simulink model "Ventilator_Controller"  (R2019b)
settings: Solver=ode23tb  StartTime=0  StopTime=1000  FixedStep=0.001  MaxStep=time_step_new  RelTol=0.01  EnableMultiTasking=on
values from neighbouring files (symbols this model uses):
  A = 20.9    [Gas_Exchange_IC.m]    (also in getPneumonia.m = (LF1-LF2)/(1-exp(Rresolve*(t2(end)-t2(1)))))
  a1 = 0.3836    [Dissociation_Spencer_IC.m]    (also in Gas_Exchange_IC.m; Respiratory_IC.m)
  a2 = 1.819    [Dissociation_Spencer_IC.m]    (also in Gas_Exchange_IC.m; Respiratory_IC.m)
  alpha1 = 0.02598    [Dissociation_Spencer_IC.m]    (also in Gas_Exchange_IC.m; Respiratory_IC.m)
  alpha2 = 0.05591    [Dissociation_Spencer_IC.m]    (also in Gas_Exchange_IC.m; Respiratory_IC.m)
  B = 92.8    [Gas_Exchange_IC.m]    (also in getPneumonia.m = LungFunction(end)-A)
  beta1 = 0.012275    [Dissociation_Spencer_IC.m]    (also in Gas_Exchange_IC.m; Respiratory_IC.m)
  beta2 = 0.03255    [Dissociation_Spencer_IC.m]    (also in Gas_Exchange_IC.m; Respiratory_IC.m)
  C = 10570    [Gas_Exchange_IC.m]
  C1 = 9    [Dissociation_Spencer_IC.m]    (also in Gas_Exchange_IC.m; Respiratory_IC.m)
  C2 = 87.00    (= 87)    [Dissociation_Spencer_IC.m]    (also in Gas_Exchange_IC.m; Respiratory_IC.m)
  Circadian_Period = 24    [Respiratory_IC.m]    (also in State_UA_Khoo_IC.m)
  CvCO2IC = 0.5116    [Body_Khoo_IC.m]    (also in Gas_Exchange_IC.m; Respiratory_IC.m = 0.5247)
  CvO2IC = 0.1672    [Body_Khoo_IC.m]    (also in Gas_Exchange_IC.m; Respiratory_IC.m = 0.1639)
  D = -5.251    [Gas_Exchange_IC.m]
  Dead1CO2IC = 0.1020    (= 0.102)    [Dead_Space_Khoo_IC.m]    (also in Gas_Exchange_IC.m; Respiratory_IC.m = 39.5616)
  Dead1O2IC = 149.8824    [Dead_Space_Khoo_IC.m]    (also in Gas_Exchange_IC.m; Respiratory_IC.m = 104.3637)
  Dead2CO2IC = 0.5274    [Dead_Space_Khoo_IC.m]    (also in Gas_Exchange_IC.m; Respiratory_IC.m = 39.6736)
  Dead2O2IC = 149.3923    [Dead_Space_Khoo_IC.m]    (also in Gas_Exchange_IC.m; Respiratory_IC.m = 104.2258)
  Dead3CO2IC = 2.2996    [Dead_Space_Khoo_IC.m]    (also in Gas_Exchange_IC.m; Respiratory_IC.m = 39.8127)
  Dead3O2IC = 147.3503    [Dead_Space_Khoo_IC.m]    (also in Gas_Exchange_IC.m; Respiratory_IC.m = 104.0505)
  Dead4CO2IC = 8.2293    [Dead_Space_Khoo_IC.m]    (also in Gas_Exchange_IC.m; Respiratory_IC.m = 40.0061)
  Dead4O2IC = 140.5179    [Dead_Space_Khoo_IC.m]    (also in Gas_Exchange_IC.m; Respiratory_IC.m = 103.8005)
  Dead5CO2IC = 22.0757    [Dead_Space_Khoo_IC.m]    (also in Gas_Exchange_IC.m; Respiratory_IC.m = 40.3359)
  Dead5O2IC = 124.5641    [Dead_Space_Khoo_IC.m]    (also in Gas_Exchange_IC.m; Respiratory_IC.m = 103.3579)
  DtotalIC = 0.3    [NeuroMuscular_IC.m]    (also in Respiratory_IC.m = 0.32)
  E_CW = 5    [Pleural_Schuessler_IC.m]    (also in Pmus_Flow_Younes_IC.m; Resp_Mech_IC.m; Respiratory_IC.m)
  E_L = 5    [Pleural_Schuessler_IC.m]    (also in Pmus_Flow_Younes_IC.m; Resp_Mech_IC.m; Respiratory_IC.m)
  fc = 0.4/60    (= 0.00666666666667)    [Respiratory_IC.m]    (also in State_UA_Khoo_IC.m)
  fcs_max = 47.78    [Cardiovascular_IC.m]    (also in Reflex_Ursino_IC.m)
  fcs_min = 2.52    [Cardiovascular_IC.m]    (also in Reflex_Ursino_IC.m)
  fcs_zero = 25    [Respiratory_IC.m]
  FlowIC = 0    [Pmus_Flow_Younes_IC.m]    (also in Resp_Mech_IC.m; Respiratory_IC.m)
  fp_inf = 6.3    [Respiratory_IC.m]
  fp_zero = 3.2    [Respiratory_IC.m]
  fs_inf = 2.10    (= 2.1)    [Respiratory_IC.m]
  fs_zero = 16.11    [Respiratory_IC.m]
  ftbs_min = 0.1    [Cardiovascular_IC.m]    (also in SA_Node_Ursino_IC.m)
  gc = 0.008/60    (= 0.000133333333333)    [Respiratory_IC.m]    (also in State_UA_Khoo_IC.m)
  h = 0.0183    [Brain_Khoo_IC.m]    (also in Gas_Exchange_IC.m; Respiratory_IC.m)
  HP_basal = 0.58    [Cardiovascular_IC.m]    (also in SA_Node_Ursino_IC.m)
  Ic = 45    [Gas_Exchange_IC.m]    (also in Respiratory_IC.m; Vent_Drive_Khoo_IC.m)
  IpCO2 = 38    [Gas_Exchange_IC.m]    (also in Respiratory_IC.m; Vent_Drive_Khoo_IC.m)
  IpO2 = 102.4    [Gas_Exchange_IC.m]    (also in Respiratory_IC.m; Vent_Drive_Khoo_IC.m)
  K1 = 13    [Dissociation_Spencer_IC.m]    (also in Gas_Exchange_IC.m; Respiratory_IC.m)
  K2 = 194.4    [Dissociation_Spencer_IC.m]    (also in Gas_Exchange_IC.m; Respiratory_IC.m)
  k_cs = 11.758    [Cardiovascular_IC.m]    (also in Reflex_Ursino_IC.m)
  k_p = 7.06    [Respiratory_IC.m]
  k_s = 0.07    [Respiratory_IC.m]
  lambda = 863    [Gas_Exchange_IC.m]    (also in Lungs_Khoo_IC.m; Respiratory_IC.m)
  Mech_Vent_pressure = 17    [Mech_vent_test.m]
  MRbCO2 = 0.0517    [Brain_Khoo_IC.m]    (also in Gas_Exchange_IC.m; Respiratory_IC.m)
  MRCO2 = 0.0033    [Body_Khoo_IC.m]    (also in Gas_Exchange_IC.m; Respiratory_IC.m)
  MRO2 = 0.0038    [Body_Khoo_IC.m]    (also in Gas_Exchange_IC.m; Respiratory_IC.m)
  NM_block_gain = 1    [Mech_vent_test.m]
  PACO2_delayIC = 39.6041    [Cardio_Mix_Lange_IC.m]    (also in Gas_Exchange_IC.m; Respiratory_IC.m = 40.4448)
  PaCO2firstIC = 0.2150    (= 0.215)    [Cardio_Mix_Lange_IC.m]    (also in Gas_Exchange_IC.m; Respiratory_IC.m = -0.2465)
  PACO2IC = 37.1484    [Gas_Exchange_IC.m]    (also in Lungs_Khoo_IC.m; Respiratory_IC.m = 40.9432)
  PaCO2secondIC = 38.4577    [Cardio_Mix_Lange_IC.m]    (also in Gas_Exchange_IC.m; Respiratory_IC.m = 40.3928)
  PAO2_delayIC = 103.8436    [Cardio_Mix_Lange_IC.m]    (also in Gas_Exchange_IC.m; Respiratory_IC.m = 103.1223)
  PaO2firstIC = -0.2838    [Cardio_Mix_Lange_IC.m]    (also in Gas_Exchange_IC.m; Respiratory_IC.m = 0.3557)
  PAO2IC = 107.1983    [Gas_Exchange_IC.m]    (also in Lungs_Khoo_IC.m; Respiratory_IC.m = 102.5153)
  PaO2secondIC = 105.4828    [Cardio_Mix_Lange_IC.m]    (also in Gas_Exchange_IC.m; Respiratory_IC.m = 103.1435)
  PbCO2IC = 48.2858    [Brain_Khoo_IC.m]    (also in Gas_Exchange_IC.m; Respiratory_IC.m = 48.5383)
  PICO2 = 0    [Dead_Space_Khoo_IC.m]    (also in Gas_Exchange_IC.m; Respiratory_IC.m)
  PICO2_change = 0    [Respiratory_IC.m]
  PIO2 = 150    [Dead_Space_Khoo_IC.m]    (also in Gas_Exchange_IC.m; Respiratory_IC.m)
  PIO2_change = -90    [Mech_vent_test.m]    (also in Respiratory_IC.m = 0)
  Pn = 90    [Cardiovascular_IC.m]    (also in Reflex_Ursino_IC.m)
  Pt_frcIC1 = 0    [Pmus_Flow_Younes_IC.m]    (also in Resp_Mech_IC.m; Respiratory_IC.m)
  Pt_frcIC2 = 0    [Pmus_Flow_Younes_IC.m]    (also in Resp_Mech_IC.m; Respiratory_IC.m)
  QdBo = 0.8333    [Brain_Khoo_IC.m]    (also in Gas_Exchange_IC.m; Respiratory_IC.m)
  R_AW = 1.27    [Pleural_Schuessler_IC.m]    (also in Pmus_Flow_Younes_IC.m; Resp_Mech_IC.m; Respiratory_IC.m)
  R_CW = 1.03    [Pleural_Schuessler_IC.m]    (also in Pmus_Flow_Younes_IC.m; Resp_Mech_IC.m; Respiratory_IC.m)
  R_L = 1.69    [Pleural_Schuessler_IC.m]    (also in Pmus_Flow_Younes_IC.m; Resp_Mech_IC.m; Respiratory_IC.m)
  RC = 0.06    [Pleural_Schuessler_IC.m]    (also in Pmus_Flow_Younes_IC.m; Resp_Mech_IC.m; Respiratory_IC.m)
  rc = 0.2/60    (= 0.00333333333333)    [Respiratory_IC.m]    (also in State_UA_Khoo_IC.m)
  SbCO2 = 0.3600    (= 0.36)    [Brain_Khoo_IC.m]    (also in Gas_Exchange_IC.m; Respiratory_IC.m)
  SCO2 = 0.0043    [Brain_Khoo_IC.m]    (also in Gas_Exchange_IC.m; Respiratory_IC.m)
  SWAo = 0.007    [Respiratory_IC.m]    (also in State_UA_Khoo_IC.m)
  T1 = 1    [Cardio_Mix_Lange_IC.m]    (also in Gas_Exchange_IC.m; Respiratory_IC.m)
  T2 = 2    [Cardio_Mix_Lange_IC.m]    (also in Gas_Exchange_IC.m; Respiratory_IC.m)
  t_CO2_duration = 0    [Respiratory_IC.m]
  t_CO2_start = 0    [Respiratory_IC.m]
  t_end_new = 4*24*60*60    (= 345600)    [Mech_vent_test.m]
  t_end_UA = 0    [Respiratory_IC.m]    (also in State_UA_Khoo_IC.m)
  t_Mech_Vent_duration = 0    [Mech_vent_test.m]
  t_Mech_Vent_start = 0    [Mech_vent_test.m]
  t_Mueller_duration = 0    [NeuroMuscular_IC.m]
  t_Mueller_insp = 0    [NeuroMuscular_IC.m]
  t_Mueller_start = 0    [NeuroMuscular_IC.m]
  t_NM_block_duration = 0    [Mech_vent_test.m]
  t_NM_block_start = 0    [Mech_vent_test.m]
  t_O2_duration = 0    [Mech_vent_test.m]    (also in Respiratory_IC.m)
  t_O2_start = 0    [Mech_vent_test.m]    (also in Respiratory_IC.m)
  t_start_new = 0    [Mech_vent_test.m]
  t_start_UA = 0    [Respiratory_IC.m]    (also in State_UA_Khoo_IC.m)
  t_valsalva_duration = 0    [NeuroMuscular_IC.m]
  t_valsalva_insp = 0    [NeuroMuscular_IC.m]
  t_valsalva_start = 0    [NeuroMuscular_IC.m]
  time_step = time_step    [acquire_data.m]    (also in acquire_data_save.m)
  VC = 5    [Pmus_Flow_Younes_IC.m]    (also in Resp_Mech_IC.m; Respiratory_IC.m)
  Vdead1 = 0.03    [Dead_Space_Khoo_IC.m]    (also in Gas_Exchange_IC.m; Respiratory_IC.m)
  Vdead2 = 0.03    [Dead_Space_Khoo_IC.m]    (also in Gas_Exchange_IC.m; Respiratory_IC.m)
  Vdead3 = 0.03    [Dead_Space_Khoo_IC.m]    (also in Gas_Exchange_IC.m; Respiratory_IC.m)
  Vdead4 = 0.03    [Dead_Space_Khoo_IC.m]    (also in Gas_Exchange_IC.m; Respiratory_IC.m)
  Vdead5 = 0.03    [Dead_Space_Khoo_IC.m]    (also in Gas_Exchange_IC.m; Respiratory_IC.m)
  Ventilator_rate = 12    [Mech_vent_test.m]
  VTCO2 = 15    [Body_Khoo_IC.m]    (also in Gas_Exchange_IC.m; Respiratory_IC.m)
  VtIC = 0    [Pmus_Flow_Younes_IC.m]    (also in Resp_Mech_IC.m; Respiratory_IC.m)
  VTO2 = 6    [Body_Khoo_IC.m]    (also in Gas_Exchange_IC.m; Respiratory_IC.m)
  Z = 0.0227    [Dissociation_Spencer_IC.m]    (also in Gas_Exchange_IC.m; Respiratory_IC.m)
undefined symbols (not defined in the file or in its folder): A_0_ua, alpha_E_FFA_Heart, alpha_E_FFA_muscle, alpha_E_GLC_Heart, alpha_E_GLC_muscle, alpha_E_GLY_muscle, alpha_E_PYR_muscle, alpha_E_TGL_adipose, alpha_E_TGL_GI, alpha_E_TGL_Heart, alpha_E_TGL_muscle, Arousal_UAIC, C_ua_awake, Cbp, Cbv, Ce_0, Cep, Cev, Chp, Chv, Cla, Clamp_class, Cmp, Cmv, Cpa, CPAP_pressure, Cpp, Cpv, Cra, Csa, Csp, Csv, CvbO2_n, CvhO2_n, CvmO2_n, DAY, delay, DietBlock, Dx, Fb, fchemo_max, fchemo_min, fchemoIC, flsIC, Ftas_I0, ftas_min, ftas_r0, FVC_activation, gain_E, Gamma, Gas_sleep, Gas_sleepM, Gb, Gblock, GbO2, Gbs_sleep, gcc_sa, gcc_sb, gcc_sp, Gclamp ... (+147)
libraries: simulink x4, simulink_extras x2
(part 8 of 8)

== system Ventilator_Controller/Respiratory System/Gas Exchange/DEAD SPACE/CO2 DEAD SPACE/Pd(2)CO2 ==
  Pd(1)CO2 : Inport
  Flow : Inport  Port=2
  Pd(3)CO2 : Inport  Port=3
  1/Vdead2 : Gain  Gain=1/Vdead2  SaturateOnIntegerOverflow=on  OutDataTypeStr=Inherit: Same as input  ParamDataTypeStr=Inherit: Same as input
  Abs (v.t) : Abs  SaturateOnIntegerOverflow=on
  Integrator : Integrator  InitialCondition=Dead2CO2IC
  Product : Product  SaturateOnIntegerOverflow=on  InputSameDT=on  OutDataTypeStr=Inherit: Same as first input
  Sum : Sum  Inputs=-+  SaturateOnIntegerOverflow=on  InputSameDT=on  OutDataTypeStr=Inherit: Same as first input
  Switch : Switch  SaturateOnIntegerOverflow=on  InputSameDT=on
  Pd(2)CO2 : Outport
  tag scope: Dead2CO2IC=global
  wires:
  Integrator/1 -> Pd(2)CO2/1, Sum/1, [Dead2CO2IC]
  Abs (v.t)/1 -> Product/2
  Flow/1 -> Abs (v.t)/1, Switch/2
  Pd(3)CO2/1 -> Switch/3
  Pd(1)CO2/1 -> Switch/1
  Sum/1 -> Product/1
  1/Vdead2/1 -> Integrator/1
  Product/1 -> 1/Vdead2/1
  Switch/1 -> Sum/2

== system Ventilator_Controller/Respiratory System/Gas Exchange/DEAD SPACE/CO2 DEAD SPACE/Pd(3)CO2 ==
  Pd(2)CO2 : Inport
  Flow : Inport  Port=2
  Pd(4)CO2 : Inport  Port=3
  1/Vdead3 : Gain  Gain=1/Vdead3  SaturateOnIntegerOverflow=on  OutDataTypeStr=Inherit: Same as input  ParamDataTypeStr=Inherit: Same as input
  Abs (v.t) : Abs  SaturateOnIntegerOverflow=on
  Integrator : Integrator  InitialCondition=Dead3CO2IC
  Product : Product  SaturateOnIntegerOverflow=on  InputSameDT=on  OutDataTypeStr=Inherit: Same as first input
  Sum : Sum  Inputs=-+  SaturateOnIntegerOverflow=on  InputSameDT=on  OutDataTypeStr=Inherit: Same as first input
  Switch : Switch  SaturateOnIntegerOverflow=on  InputSameDT=on
  Pd(3)CO2 : Outport
  tag scope: Dead3CO2IC=global
  wires:
  Abs (v.t)/1 -> Product/2
  Flow/1 -> Abs (v.t)/1, Switch/2
  Switch/1 -> Sum/2
  Product/1 -> 1/Vdead3/1
  1/Vdead3/1 -> Integrator/1
  Integrator/1 -> Sum/1, Pd(3)CO2/1, [Dead3CO2IC]
  Sum/1 -> Product/1
  Pd(2)CO2/1 -> Switch/1
  Pd(4)CO2/1 -> Switch/3

== system Ventilator_Controller/Respiratory System/Gas Exchange/DEAD SPACE/CO2 DEAD SPACE/Pd(4)CO2 ==
  Pd(3)CO2 : Inport
  Flow : Inport  Port=2
  Pd(5)CO2 : Inport  Port=3
  1/Vdead4 : Gain  Gain=1/Vdead4  SaturateOnIntegerOverflow=on  OutDataTypeStr=Inherit: Same as input  ParamDataTypeStr=Inherit: Same as input
  Abs (v.t) : Abs  SaturateOnIntegerOverflow=on
  Integrator : Integrator  InitialCondition=Dead4CO2IC
  Product : Product  SaturateOnIntegerOverflow=on  InputSameDT=on  OutDataTypeStr=Inherit: Same as first input
  Sum : Sum  Inputs=-+  SaturateOnIntegerOverflow=on  InputSameDT=on  OutDataTypeStr=Inherit: Same as first input
  Switch : Switch  SaturateOnIntegerOverflow=on  InputSameDT=on
  Pd(4)CO2 : Outport
  tag scope: Dead4CO2IC=global
  wires:
  Abs (v.t)/1 -> Product/2
  Flow/1 -> Abs (v.t)/1, Switch/2
  Pd(5)CO2/1 -> Switch/3
  Pd(3)CO2/1 -> Switch/1
  Sum/1 -> Product/1
  1/Vdead4/1 -> Integrator/1
  Product/1 -> 1/Vdead4/1
  Switch/1 -> Sum/2
  Integrator/1 -> Pd(4)CO2/1, [Dead4CO2IC], Sum/1

== system Ventilator_Controller/Respiratory System/Gas Exchange/DEAD SPACE/CO2 DEAD SPACE/Pd(5)CO2 ==
  Pd(4)CO2 : Inport
  Flow : Inport  Port=2
  PACO2 : Inport  Port=3
  1/Vdead5 : Gain  Gain=1/Vdead5  SaturateOnIntegerOverflow=on  OutDataTypeStr=Inherit: Same as input  ParamDataTypeStr=Inherit: Same as input
  Abs (v.t) : Abs  SaturateOnIntegerOverflow=on
  Integrator : Integrator  InitialCondition=Dead5CO2IC
  Product : Product  SaturateOnIntegerOverflow=on  InputSameDT=on  OutDataTypeStr=Inherit: Same as first input
  Sum : Sum  Inputs=-+  SaturateOnIntegerOverflow=on  InputSameDT=on  OutDataTypeStr=Inherit: Same as first input
  Switch : Switch  SaturateOnIntegerOverflow=on  InputSameDT=on
  Pd(5)CO2 : Outport
  tag scope: Dead5CO2IC=global
  wires:
  Abs (v.t)/1 -> Product/2
  Flow/1 -> Abs (v.t)/1, Switch/2
  Switch/1 -> Sum/2
  Product/1 -> 1/Vdead5/1
  1/Vdead5/1 -> Integrator/1
  Integrator/1 -> Sum/1, Pd(5)CO2/1, [Dead5CO2IC]
  Sum/1 -> Product/1
  Pd(4)CO2/1 -> Switch/1
  PACO2/1 -> Switch/3

== system Ventilator_Controller/Respiratory System/Gas Exchange/DEAD SPACE/O2 DEAD SPACE/Pd(1)O2 ==
  PIO2 : Inport
  Flow : Inport  Port=2
  Pd(2)O2 : Inport  Port=3
  1/Vdead1 : Gain  Gain=1/Vdead1  SaturateOnIntegerOverflow=on  OutDataTypeStr=Inherit: Same as input  ParamDataTypeStr=Inherit: Same as input
  Abs (v.t) : Abs  SaturateOnIntegerOverflow=on
  Integrator : Integrator  InitialCondition=Dead1O2IC
  Product : Product  SaturateOnIntegerOverflow=on  InputSameDT=on  OutDataTypeStr=Inherit: Same as first input
  Sum : Sum  Inputs=-+  SaturateOnIntegerOverflow=on  InputSameDT=on  OutDataTypeStr=Inherit: Same as first input
  Switch : Switch  SaturateOnIntegerOverflow=on  InputSameDT=on
  Pd(1)O2 : Outport
  tag scope: Dead1O2IC=global
  wires:
  Switch/1 -> Sum/2
  Pd(2)O2/1 -> Switch/3
  PIO2/1 -> Switch/1
  Sum/1 -> Product/1
  Integrator/1 -> Sum/1, Pd(1)O2/1, [Dead1O2IC]
  1/Vdead1/1 -> Integrator/1
  Product/1 -> 1/Vdead1/1
  Flow/1 -> Abs (v.t)/1, Switch/2
  Abs (v.t)/1 -> Product/2

== system Ventilator_Controller/Respiratory System/Gas Exchange/DEAD SPACE/O2 DEAD SPACE/Pd(2)O2 ==
  Pd(1)O2 : Inport
  Flow : Inport  Port=2
  Pd(3)O2 : Inport  Port=3
  1/Vdead2 : Gain  Gain=1/Vdead2  SaturateOnIntegerOverflow=on  OutDataTypeStr=Inherit: Same as input  ParamDataTypeStr=Inherit: Same as input
  Abs (v.t) : Abs  SaturateOnIntegerOverflow=on
  Integrator : Integrator  InitialCondition=Dead2O2IC
  Product : Product  SaturateOnIntegerOverflow=on  InputSameDT=on  OutDataTypeStr=Inherit: Same as first input
  Sum : Sum  Inputs=-+  SaturateOnIntegerOverflow=on  InputSameDT=on  OutDataTypeStr=Inherit: Same as first input
  Switch : Switch  SaturateOnIntegerOverflow=on  InputSameDT=on
  Pd(2)O2 : Outport
  tag scope: Dead2O2IC=global
  wires:
  Abs (v.t)/1 -> Product/2
  Flow/1 -> Abs (v.t)/1, Switch/2
  Product/1 -> 1/Vdead2/1
  Integrator/1 -> [Dead2O2IC], Sum/1, Pd(2)O2/1
  Sum/1 -> Product/1
  Pd(1)O2/1 -> Switch/1
  Pd(3)O2/1 -> Switch/3
  Switch/1 -> Sum/2
  1/Vdead2/1 -> Integrator/1

== system Ventilator_Controller/Respiratory System/Gas Exchange/DEAD SPACE/O2 DEAD SPACE/Pd(3)O2 ==
  Pd(2)O2 : Inport
  Flow : Inport  Port=2
  Pd(4)O2 : Inport  Port=3
  1/Vdead3 : Gain  Gain=1/Vdead3  SaturateOnIntegerOverflow=on  OutDataTypeStr=Inherit: Same as input  ParamDataTypeStr=Inherit: Same as input
  Abs (v.t) : Abs  SaturateOnIntegerOverflow=on
  Integrator : Integrator  InitialCondition=Dead3O2IC
  Product : Product  SaturateOnIntegerOverflow=on  InputSameDT=on  OutDataTypeStr=Inherit: Same as first input
  Sum : Sum  Inputs=-+  SaturateOnIntegerOverflow=on  InputSameDT=on  OutDataTypeStr=Inherit: Same as first input
  Switch : Switch  SaturateOnIntegerOverflow=on  InputSameDT=on
  Pd(3)O2 : Outport
  tag scope: Dead3O2IC=global
  wires:
  Switch/1 -> Sum/2
  Pd(4)O2/1 -> Switch/3
  Pd(2)O2/1 -> Switch/1
  Sum/1 -> Product/1
  Integrator/1 -> [Dead3O2IC], Sum/1, Pd(3)O2/1
  Product/1 -> 1/Vdead3/1
  Flow/1 -> Abs (v.t)/1, Switch/2
  Abs (v.t)/1 -> Product/2
  1/Vdead3/1 -> Integrator/1

== system Ventilator_Controller/Respiratory System/Gas Exchange/DEAD SPACE/O2 DEAD SPACE/Pd(4)O2 ==
  Pd(3)O2 : Inport
  Flow : Inport  Port=2
  Pd(5)O2 : Inport  Port=3
  1/Vdead4 : Gain  Gain=1/Vdead4  SaturateOnIntegerOverflow=on  OutDataTypeStr=Inherit: Same as input  ParamDataTypeStr=Inherit: Same as input
  Abs (v.t) : Abs  SaturateOnIntegerOverflow=on
  Integrator : Integrator  InitialCondition=Dead4O2IC
  Product : Product  SaturateOnIntegerOverflow=on  InputSameDT=on  OutDataTypeStr=Inherit: Same as first input
  Sum : Sum  Inputs=-+  SaturateOnIntegerOverflow=on  InputSameDT=on  OutDataTypeStr=Inherit: Same as first input
  Switch : Switch  SaturateOnIntegerOverflow=on  InputSameDT=on
  Pd(4)O2 : Outport
  tag scope: Dead4O2IC=global
  wires:
  Abs (v.t)/1 -> Product/2
  Flow/1 -> Abs (v.t)/1, Switch/2
  Product/1 -> 1/Vdead4/1
  Integrator/1 -> Sum/1, Pd(4)O2/1, [Dead4O2IC]
  Sum/1 -> Product/1
  Pd(3)O2/1 -> Switch/1
  Pd(5)O2/1 -> Switch/3
  Switch/1 -> Sum/2
  1/Vdead4/1 -> Integrator/1

== system Ventilator_Controller/Respiratory System/Gas Exchange/DEAD SPACE/O2 DEAD SPACE/Pd(5)O2 ==
  Pd(4)O2 : Inport
  Flow : Inport  Port=2
  PAO2 : Inport  Port=3
  1/Vdead5 : Gain  Gain=1/Vdead5  SaturateOnIntegerOverflow=on  OutDataTypeStr=Inherit: Same as input  ParamDataTypeStr=Inherit: Same as input
  Abs (v.t) : Abs  SaturateOnIntegerOverflow=on
  Integrator : Integrator  InitialCondition=Dead5O2IC
  Product : Product  SaturateOnIntegerOverflow=on  InputSameDT=on  OutDataTypeStr=Inherit: Same as first input
  Sum : Sum  Inputs=-+  SaturateOnIntegerOverflow=on  InputSameDT=on  OutDataTypeStr=Inherit: Same as first input
  Switch : Switch  SaturateOnIntegerOverflow=on  InputSameDT=on
  Pd(5)O2 : Outport
  tag scope: Dead5O2IC=global
  wires:
  Switch/1 -> Sum/2
  PAO2/1 -> Switch/3
  Pd(4)O2/1 -> Switch/1
  Sum/1 -> Product/1
  Integrator/1 -> Pd(5)O2/1, [Dead5O2IC], Sum/1
  Product/1 -> 1/Vdead5/1
  Flow/1 -> Abs (v.t)/1, Switch/2
  Abs (v.t)/1 -> Product/2
  1/Vdead5/1 -> Integrator/1

== system Ventilator_Controller/Respiratory System/Gas Exchange/DEAD SPACE/CO2 DEAD SPACE/CO2 Partial Pressure/If Action Subsystem ==
  In1 : Inport
  In2 : Inport  Port=2
  Action Port : ActionPort  ActionPortLabel=if(u1 > 38.87)
  Integrator : Integrator
  Product1 : Product  RndMeth=Zero
  Out1 : Outport  InitialOutput=0
  wires:
  Product1/1 -> Integrator/1
  In2/1 -> Product1/2
  In1/1 -> Product1/1
  Integrator/1 -> Out1/1

== system Ventilator_Controller/Respiratory System/Gas Exchange/DEAD SPACE/CO2 DEAD SPACE/CO2 Partial Pressure/If Action Subsystem1 ==
  In1 : Inport
  In2 : Inport  Port=2
  Action Port : ActionPort  ActionPortLabel=elseif(u1<38.7)
  Integrator : Integrator
  Product1 : Product  RndMeth=Zero
  Out1 : Outport  InitialOutput=0
  wires:
  Product1/1 -> Integrator/1
  In2/1 -> Product1/2
  In1/1 -> Product1/1
  Integrator/1 -> Out1/1

== matlab function Ventilator_Controller/Respiratory System/Sleep Mechanism/Embedded MATLAB Function1 ==
  data: t0 input; u2 input; y output; t input
function y = fcn(t0, u2, t)
% This block supports an embeddable subset of the MATLAB language.
% See the help menu for details. 

% day = floor(para/3600/24);
% t0 = 0;
% count = 0;
% while count <=day
% if u1>0.5 %sleep/awake state change
%     t0 = t
% end
if u2 <0.5 %sleep start %sleep/awake state change
    y=0;
else %u2 >0.5 %(awake state)
    if (t>= t0 + 1.5*3600+5) && (t <= t0 + 1.5*3600+15*60+5)   %Breakfast
%     if (t>= t0 + 2*3600+5) && (t <= t0 + 2*3600+15*60+5)   %Breakfast
        y=22/60;
    elseif (t>= t0 + 5.5*3600+5) && (t <= t0 + 5.5*3600+30*60+5)%Lunch
        y=30/60;
    elseif (t>= t0 + 12*3600+5) && (t <=t0 + 12*3600+45*60+5)%dinner
        y=24/60;
    else %NREMs
        y=0; 
    end

end

== matlab function Ventilator_Controller/Metabolic Control/Glucose Insulin Interventions/Hyper//Eu//Hypo glycemic Clamp (step by step)/Embedded MATLAB Function ==
  data: t input; y output; Gb_clamp input; Gt input; t0 input; Gt1 input; PFGinf input; meta output; meta2 input
function [y,meta]  = fcn(t,Gb_clamp,Gt,t0,Gt1,PFGinf,meta2)
% This block supports the Embedded MATLAB subset.
% See the help menu for details. 
% PF=117*96*3;%1.3;%with 117*1.2 same as 117*1.3, reach 235-116=119 at steady state%VolG
% Ginf=2;
% if t>=t0(1) && t<(t0(1)+15*60) %first 15 minute priming dose
% %     if Gt<= (Gb_clamp(1)+Gb_clamp(2))
% %         y=t-t0(1);
% %         meta=0;
% %     else
% %         meta = meta2*(Gb_clamp(2)/(Gt-Gb_clamp(1)))*(Gb_clamp(2)/(Gt1-Gb_clamp(1)));
% %         y=(Gb_clamp(1)+Gb_clamp(2)-Gt)*10*0.19*70/(Ginf*15*60)*PF +meta*4;%bodywt=70
% 
%         y=46.455;%with 47,reach 242-116=126 at the end of 15 minute%45;20/4;
%         meta=0;
% %     end
% factor =1/SurfaceArea;%6;%240/47*1.5;
% sec=1;%minute to second 60
% meta=1;
% if t>=t0(1) && t<(t0(1)+1*sec)
%     y=1768/factor;%with 47,reach 242-116=126 at the end of 15 minute%45;20/4;
%     meta=1;
% elseif t>=(t0(1)+1*sec) && t<(t0(1)+2*sec)
%     y=1428/factor;%with 47,reach 242-116=126 at the end of 15 minute%45;20/4;
%     meta=1;
% elseif t>=(t0(1)+2*sec) && t<(t0(1)+3*sec)
%     y=1156/factor;%with 47,reach 242-116=126 at the end of 15 minute%45;20/4;
%     meta=1;
% elseif t>=(t0(1)+3*sec) && t<(t0(1)+4*sec)
%     y=918/factor;%with 47,reach 242-116=126 at the end of 15 minute%45;20/4;
%     meta=1;
% elseif t>=(t0(1)+4*sec) && t<(t0(1)+5*sec)
%     y=782/factor;%with 47,reach 242-116=126 at the end of 15 minute%45;20/4;
%     meta=1;
% elseif t>=(t0(1)+5*sec) && t<(t0(1)+6*sec)
%     y=646/factor;%with 47,reach 242-116=126 at the end of 15 minute%45;20/4;
%     meta=1;
% elseif t>=(t0(1)+6*sec) && t<(t0(1)+7*sec)
%     y=544/factor;%with 47,reach 242-116=126 at the end of 15 minute%45;20/4;
%     meta=1;
% elseif t>=(t0(1)+7*sec) && t<(t0(1)+8*sec)
%     y=442/factor;%with 47,reach 242-116=126 at the end of 15 minute%45;20/4;
%     meta=1;
% elseif t>=(t0(1)+8*sec) && t<(t0(1)+9*sec)
%     y=408/factor;%with 47,reach 242-116=126 at the end of 15 minute%45;20/4;
%     meta=1;
% elseif t>=(t0(1)+9*sec) && t<(t0(1)+10*sec)
%     y=374/factor;%with 47,reach 242-116=126 at the end of 15 minute%45;20/4;
%     meta=1;
% elseif t>=(t0(1)+10*sec) && t<(t0(1)+11*60)
%     y=340/factor;%with 47,reach 242-116=126 at the end of 15 minute%45;20/4;
%     meta=1;
% elseif t>=(t0(1)+11*sec) && t<(t0(1)+12*sec)
%     y=306/factor;%with 47,reach 242-116=126 at the end of 15 minute%45;20/4;
%     meta=1;
% elseif t>=(t0(1)+12*sec) && t<(t0(1)+13*sec)
%     y=272/factor;%with 47,reach 242-116=126 at the end of 15 minute%45;20/4;
%     meta=1;
% elseif t>=(t0(1)+13*sec) && t<(t0(1)+14*sec)
%     y=238/factor;%with 47,reach 242-116=126 at the end of 15 minute%45;20/4;
%     meta=1;
% elseif t>= (t0(1)+14*sec) && t<t0(2)% maintenace dose
y=0;
meta=0;
if t>t0(1)&& t<t0(2)
    if Gb_clamp(2)>0
        meta = meta2*(Gb_clamp(2)/(Gt-Gb_clamp(1)))*(Gb_clamp(2)/(Gt1-Gb_clamp(1)));
    else
        meta = meta2*(Gb_clamp(1)/Gt)*(Gb_clamp(1)/Gt1);
    end
%     y=meta;
    y=(Gb_clamp(1)+Gb_clamp(2)-Gt)*10*0.19*70/15*PFGinf +meta;%bodywt=70
%this condition will cause huge oscillations for metabolic component
% elseif t==t0(1)
%     y = 0;
%     meta=4*70;
else
    y=0;
    if Gb_clamp(2)>0
        meta=28*70/60;
    else
        meta=0.5*70/60;%4*70;
    end
%     meta=1/60;%/60;
end

== matlab function Ventilator_Controller/Respiratory System/Sleep Mechanism/Embedded MATLAB Function ==
  data: t0 input; u2 input; y output; t input
function y = fcn(t0, u2, t)
% This block supports an embeddable subset of the MATLAB language.
% See the help menu for details. 

% day = floor(para/3600/24);
% t0 = 0;
% count = 0;
% while count <=day
% if u1>0.5 %sleep/awake state change
%     t0 = t
% end
if u2 >0.5 %awake state %sleep/awake state change
    y=0;
else %u2 <0.5 %(sleep start)
    if (t>=t0 + 0.85*1.8*3600+5) && (t <=t0 + 1*1.8*3600+5)   %1st REM
        y=1;
    elseif (t>=t0 + (1+0.85)*1.8*3600+5) && (t <=t0 + 2*1.8*3600+5)%2nd REM
        y=1;
    elseif (t>=t0 + (2+0.85)*1.8*3600+5) && (t <=t0 + 3*1.8*3600+5)%3rd REM
        y=1;
    elseif (t>=t0 + (3+0.85)*1.8*3600+5) && (t <=t0 + 4*1.8*3600+5)%4 REM
        y=1;
    elseif (t>=t0 + (4+0.85)*1.8*3600+5) && (t <=t0 + 5*1.8*3600+5)%5 REM
        y=1;
    elseif (t>=t0 + (5+0.85)*1.8*3600+5) && (t <=t0 + 6*1.8*3600+5)%6 REM
        y=1;
    else %NREMs
        y=0; 
    end

end
